simulink library "lib_lowphy"  (R2023b)
settings: Solver=VariableStepAuto  StartTime=0.0  StopTime=10.0  RelTol=1e-3
undefined symbols (not defined in the file or in its folder): AdvDSPBChannelOutDisplay, AdvDSPBDMemDisplay, AdvDSPBInDisplay, AdvDSPBOutDisplay, dpoly, dspba, dspba_ChannelInVis, dspba_ChannelOutVis, dspba_internal_get_channel_ports, evalAionMaskParam, fft_tb_in, ifft_tb_in, latency, latencyCorrection, max_FFTStages, max_NSubcarriers, primtype, UseDontCare, value
libraries: DSPBAPrim x637, DSPBAControl x55, $bdroot x16, DSPBAModelBus x12, DSPBAUtilities x6, DSPBABase x5, DSPBAWaveformSynth x4, DspbAdvFftLibrary x3, DSPBAVectorUtil x2, DspbAdvVfftPrefix x1
(part 1 of 9)
settings Model: Creator=manjukri  LastModifiedBy=5g
settings DebuggingCC: UnconnectedInputMsg=warning  UnconnectedOutputMsg=warning  UnconnectedLineMsg=warning
settings ModelReferenceCC: EnableRefExpFcnMdlSchedulingChecks=on
settings RTWCC: DLArmComputeVersion=19.05

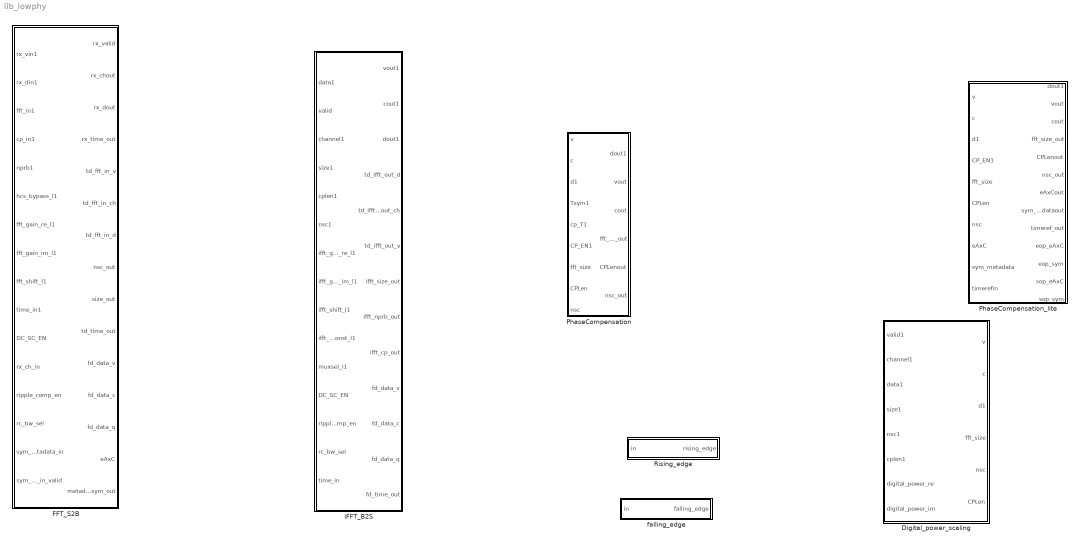
== system lib_lowphy ==
  Digital_power_scaling : Subsystem
  FFT_S2B : Subsystem  mask{FFTmaxsize=12, FFTminsize=9, FFTstages=12, Rx_scaling=2^-12, AxCdelay=288, NCO_addr_offset=0, rc_out_frac=11}
      mask prompts: FFTmaxsize "FFT max size"; FFTminsize "FFT Min Size"; FFTstages "FFT stages"; Rx_scaling "Fractional Precision output of FFT"; AxCdelay "delay between AxC block output"; NCO_addr_offset "NCO address offset (length =4)"; rc_out_frac "enter_ripple_comp_out_frac_bits"
      mask init:
      | fsmpaths
      | 
      | 
      | 
      | 
      | %% FFT configuration
      | dspb_fft_multichannel.IFFT = false;
      | dspb_fft_multichannel.minsize = FFTminsize;
      | dspb_fft_multichannel.maxsize = FFTmaxsize;
      | dspb_fft_multichannel.N = FFTstages;
      | dspb_fft_multichannel.subchannels = 1; % must be a power of 2
      | dspb_fft_multichannel.FFTsize = 2^dspb_fft_multichannel.N;
      | dspb_fft_multichannel.blockSize = dspb_fft_multichannel.subchannels * dspb_fft_multichannel.FFTsize;
      | 
      | %% Data widths
      | dspb_fft_multichannel.InputType   = fixdt(1,16,13);
      | dspb_fft_multichannel.TwiddleType = fixdt(1,16,15);
      | 
      | dspb_fft_multichannel.Phase_Inversion_l1   = 15;
      | dspb_fft_multichannel.fft_gain_offset_l1   = 1;
      | dspb_fft_multichannel.fft_gain_value       = 1;
      | dspb_fft_multichannel.HCS_Bypass_offset_l1 = 2;
      | dspb_fft_multichannel.HCS_Bypass_value     = 1;
      | 
      | dspb_fft_multichannel.Phase_Inversion_l2   = 20;
      | dspb_fft_multichannel.fft_gain_offset_l2   = 3;
      | dspb_fft_multichannel.HCS_Bypass_offset_l2 = 4;
      | dspb_fft_multichannel.sclowerselect_l2 =5;
      | dspb_fft_multichannel.ClockRate	=  491.52;
      | 
      | 
      | %% Pruning options
      | %dspb_fft_multichannel.TypeStrings0 = some user-defined strategy
      | 
      | dspb_fft_multichannel.TypeStrings1 = ...
      |     dspba.fft.full_wordgrowth(true, false, dspb_fft_multichannel.N,...
      |         dspb_fft_multichannel.InputType, dspb_fft_multichannel.TwiddleType);
      | 
      | dspb_fft_multichannel.TypeStrings2 = ...
      |     dspba.fft.mild_pruning(true, false, dspb_fft_multichannel.N,...
      |         dspb_fft_multichannel.InputType, dspb_fft_multichannel.TwiddleType); 
      | 
      | dspb_fft_multichannel.TypeStrings3 = ...
      |     dspba.fft.prune_to_width(19, true, false, dspb_fft_multichannel.N,...
      |         dspb_fft_multichannel.InputType, dspb_fft_multichannel.TwiddleType);
      | 
      | dspb_fft_multichannel.TypeStrings = dspb_fft_multichannel.TypeStrings1;
      | 
      | 
      | 
      | FeedbackDelay1=12;
  PhaseCompensation : Subsystem  mask{Tc=1/122.88e6, CP_1=352, CP_2=288, PhaseGen_TXRX=0, Op_frac_scaling=2^-14}
      mask prompts: Tc "Sample time"; CP_1 "CP Sample Length Sym 0"; CP_2 "CP Sample Length Sym 1-13"; PhaseGen_TXRX "Phase Sign (1= -ve phase for Tx , 0 = +ve phase for Rx)"; Op_frac_scaling "Output Fractional scaling"
      mask init:
      | %% MM Register Setting
      | MMoffset.F1_regLSB = 0;
      | MMoffset.F1_regMSB = 1;
      | MMoffset.Enable_reg1 = 2;
      | MMoffset.PhaseGen_reg = 3;
      | 
      | 
      | 
      | 
      | cordic_gain = 1.646760257865452963193594414453;
      | 
      | 
      | 
      | CPSample_Vector_LUT = [ CP_1*Tc CP_2*Tc*ones(1,13)]*1e9; % t is given in ns as F is given in Ghz
      | 
      | 
      | 
      | 
      | 
      | 
      | dspb_ifft_multichannel.ClockRate=491.52;
  PhaseCompensation_lite : Subsystem  mask{Tc=1/122.88e6, CP_1=352, CP_2=288, PhaseGen_TXRX=0, Op_frac_scaling=2^-14, reg_mem_offset_rf_freq=0, reg_mem_offset_Phase_comp_enable=1, reg_mem_offset_tx_rx_sel=2}
      mask prompts: Tc "Sample time"; CP_1 "CP Sample Length Sym 0"; CP_2 "CP Sample Length Sym 1-13"; PhaseGen_TXRX "Phase Sign (1= -ve phase for Tx , 0 = +ve phase for Rx)"; Op_frac_scaling "Output Fractional scaling"; reg_mem_offset_rf_freq "Address offset of register holding RF Frequency"; reg_mem_offset_Phase_comp_enable "Address offset of register holding Phase Compensation enable"; reg_mem_offset_tx_rx_sel "Address offset of register holding  Tx Rx Selection"
      mask init:
      | %% MM Register Setting
      | MMoffset.F1_regLSB = 0;
      | MMoffset.F1_regMSB = 1;
      | MMoffset.Enable_reg1 = 2;
      | MMoffset.PhaseGen_reg = 3;
      | 
      | 
      | 
      | 
      | cordic_gain = 1.646760257865452963193594414453;
      | 
      | 
      | 
      | CPSample_Vector_LUT = [ CP_1*Tc CP_2*Tc*ones(1,13)]*1e9; % t is given in ns as F is given in Ghz
      | 
      | 
      | 
      | 
      | 
      | 
      | dspb_ifft_multichannel.ClockRate=491.52;
      | 
      | %Tsym_reinterpret_LUT=[ 2.87272135416667e-06 3.85498046875000e-05 7.42268880208333e-05 0.000109903971354167 0.000145581054687500 0.000181258138020833 0.000216935221354167 0.000252612304687500 0.000288289388020833 0.000323966471354167 0.000359643554687500 0.000395320638020833 0.000430997721354167 0.000466674804687500 ]*1e9;
  Rising_edge : Subsystem
      mask init:
      | fsmpaths
  falling_edge : Subsystem
      mask init:
      | fsmpaths
  iFFT_B2S : Subsystem  mask{iFFTmaxsize=12, iFFTminsize=9, iFFTstages=12, Tx_scaling=2^-14, Bw_Delay_en=1, rc_out_frac=12}
      mask prompts: iFFTmaxsize "iFFT Maxsize"; iFFTminsize "iFFT Minsize"; iFFTstages "iFFT Stages"; Tx_scaling "Fractional precision output of iFFT_B2B"; Bw_Delay_en "Delay Alignment for Bandwidth (60 & 100MHz)"; rc_out_frac "ripple compensation out fractional value"
      mask init:
      | %% IFFT configuration
      | dspb_ifft_multichannel.IFFT = true;
      | dspb_ifft_multichannel.minsize = iFFTminsize;
      | dspb_ifft_multichannel.maxsize = iFFTmaxsize;
      | dspb_ifft_multichannel.N = iFFTstages;
      | dspb_ifft_multichannel.subchannels = 1; % must be a power of 2
      | dspb_ifft_multichannel.FFTsize = 2^dspb_ifft_multichannel.N;
      | dspb_ifft_multichannel.blockSize = dspb_ifft_multichannel.subchannels * dspb_ifft_multichannel.FFTsize;
      | 
      | %% Data widths
      | dspb_ifft_multichannel.InputType   = fixdt(1,16,rc_out_frac);
      | dspb_ifft_multichannel.TwiddleType = fixdt(1,16,15);
      | 
      | 
      | 
      | 
      | %% Pruning options
      | %dspb_ifft_multichannel.TypeStrings0 = some user-defined strategy
      | 
      | dspb_ifft_multichannel.TypeStrings1 = ...
      |     dspba.fft.full_wordgrowth(true, false, dspb_ifft_multichannel.N,...
      |         dspb_ifft_multichannel.InputType, dspb_ifft_multichannel.TwiddleType);
      | 
      | dspb_ifft_multichannel.TypeStrings2 = ...
      |     dspba.fft.mild_pruning(true, false, dspb_ifft_multichannel.N,...
      |         dspb_ifft_multichannel.InputType, dspb_ifft_multichannel.TwiddleType);
      | 
      | dspb_ifft_multichannel.TypeStrings3 = ...
      |     dspba.fft.prune_to_width(19, true, false, dspb_ifft_multichannel.N,...
      |         dspb_ifft_multichannel.InputType, dspb_ifft_multichannel.TwiddleType);
      | 
      | dspb_ifft_multichannel.TypeStrings = dspb_ifft_multichannel.TypeStrings1;
      | 
      | %%
      |  CP_ProcessingDelay =30;
      | SampleReg_pipelineDelay = 14;
      | max_FFTStages=iFFTstages;
      | max_NSubcarriers=3276;

== system lib_lowphy/Digital_power_scaling ==
  valid1 : Inport
  channel1 : Inport  Port=2
  data1 : Inport  Port=3
  size1 : Inport  Port=4
  nsc1 : Inport  Port=5
  cplen1 : Inport  Port=6
  digital_power_re : Inport  Port=7
  digital_power_im : Inport  Port=8
  Mult : DSPBAPrim/Mult  primtype=mult  nInputs=2  nOutputs=1  omode=Inherit via internal rule  otype=sfix(16)  scale=2^-15  rndmethod=Unbiased  factor=1  satmethod=Symmetric  shift_vec=[0 1 2 -1]  value=0  inPortNames=[' '; ' ';]  outPortNames=[' ']  dspbaimage=dspba_prim.svg  text=fprintf('X');  style=Optimised  visibilities=8+2^18+2^19  floatPrecision=float32_m23  floatRounding=correct  advOptions=[]  version=20211007
  Real-Imag to Complex : RealImagToComplex
  Scale1 : DSPBAPrim/Convert  primtype=convert  nInputs=1  nOutputs=1  omode=Specify via dialog  otype=sfix(16)  scale=2^-15  rndmethod=Biased  factor=1  satmethod=Symmetric  shift_vec=[0 1 2 -1]  value=round([0:255]/17)  inPortNames=[' '; ' ';]  outPortNames=[' '; 'c']  dspbaimage=dspba_prim_wide.svg  text=fprintf('convert');  style=Optimised  visibilities=8+64+256+2^17  clipdetect=off  floatPrecision=float32_m23  advOptions=[]  version=20211007
  SynthesisInfo : DSPBAPrim/SynthesisInfo  primtype=synthinfo  nInputs=0  nOutputs=0  omode=Inherit via internal rule  otype=sfix(16)  scale=2^-15  rndmethod=Truncate  factor=1  satmethod=Symmetric  shift_vec=[0 1 2 -1]  value=99  inPortNames=[' '; ' ';]  outPortNames=[' ']  dspbaimage=dspba_prim_ctrl.jpg  text=fprintf('Style=%s', style);  style=Scheduled  visibilities=2^17+2^18+2^19+2^20+2^21+2^22+2^23+2^24  constraintPair=None  constraintRelation=>  constraintLimit=2  modelRefSign=+  modelRef=''  showSchedule=off  simulationMode=Use Global Value  resetMinimization=Conditional - On for ChannelIn/Out only  version=20220106
  channel_DPS1_in : DSPBAPrim/ChannelIn  primtype=channelin  nInputs=dspba_internal_get_channel_ports(gcb)  nOutputs=dspba_internal_get_channel_ports(gcb)  omode=Inherit via internal rule  otype=sfix(16)  scale=2^-15  rndmethod=Unbiased  factor=1  satmethod=Symmetric  shift_vec=[0 1 2 -1]  value=6  inPortNames=['v'; 'c'; '0'; '1'; '2'; '3'; '4'; '5'; '6'; '7'; '8'; '9'; 'A'; 'B'; 'D'; 'E'; 'F'; 'G'; 'H'; 'I'; 'J'; 'K'; 'L'; 'M'; 'N'; 'O'; 'P'; 'Q'; 'R'; 'S'; 'T'; 'U'; 'W'; 'X'; 'Y'; 'Z']  outPortNames=['v'; 'c'; '0'; '1'; '2'; '3'; '4'; '5'; '6'; '7'; '8'; '9'; 'A'; 'B'; 'D'; 'E'; 'F'; 'G'; 'H'; 'I'; 'J'; 'K'; 'L'; 'M'; 'N'; 'O'; 'P'; 'Q'; 'R'; 'S'; 'T'; 'U'; 'W'; 'X'; 'Y'; 'Z']  dspbaimage=dspba_prim_channel_tall.svg  text=fprintf('In');  style=Optimised  dataSignals=6  foldingEnabled=off  channels=1  sampleRate=200  packetBeginPresent=off  packetBeginEnabled=off  visibilities=dspba_ChannelInVis(gcb)  latencyCorrection=0  scheduleOrigin=on  version=20211214
  channel_DPS1_out : DSPBAPrim/ChannelOut  primtype=channelout  nInputs=dspba_internal_get_channel_ports(gcb)  nOutputs=dspba_internal_get_channel_ports(gcb)  omode=Inherit via internal rule  otype=sfix(16)  scale=2^-15  rndmethod=Unbiased  factor=1  satmethod=Symmetric  shift_vec=[0 1 2 -1]  value=4  inPortNames=['v'; 'c'; '0'; '1'; '2'; '3'; '4'; '5'; '6'; '7'; '8'; '9'; 'A'; 'B'; 'D'; 'E'; 'F'; 'G'; 'H'; 'I'; 'J'; 'K'; 'L'; 'M'; 'N'; 'O'; 'P'; 'Q'; 'R'; 'S'; 'T'; 'U'; 'W'; 'X'; 'Y'; 'Z']  outPortNames=['v'; 'c'; '0'; '1'; '2'; '3'; '4'; '5'; '6'; '7'; '8'; '9'; 'A'; 'B'; 'D'; 'E'; 'F'; 'G'; 'H'; 'I'; 'J'; 'K'; 'L'; 'M'; 'N'; 'O'; 'P'; 'Q'; 'R'; 'S'; 'T'; 'U'; 'W'; 'X'; 'Y'; 'Z']  dspbaimage=dspba_prim_channel_tall.svg  text=fprintf('Out%s', AdvDSPBChannelOutDisplay(latency));  style=Optimised  dataSignals=4  foldingEnabled=off  channels=1  sampleRate=200  packetBeginPresent=off  packetBeginEnabled=off  visibilities=dspba_ChannelOutVis(gcb)  latency=8  latencyCorrection=0  version=20211214
  v : Outport
  c : Outport  Port=2
  d1 : Outport  Port=3
  fft_size : Outport  Port=4
  nsc : Outport  Port=5
  CPLen : Outport  Port=6
  wires:
  valid1/1 -> channel_DPS1_in/1
  channel1/1 -> channel_DPS1_in/2
  data1/1 -> channel_DPS1_in/3
  channel_DPS1_out/3 -> d1/1
  channel_DPS1_out/4 -> fft_size/1
  channel_DPS1_out/2 -> c/1
  channel_DPS1_out/1 -> v/1
  size1/1 -> channel_DPS1_in/4
  nsc1/1 -> channel_DPS1_in/5
  channel_DPS1_out/5 -> nsc/1
  cplen1/1 -> channel_DPS1_in/6
  digital_power_re/1 -> channel_DPS1_in/7
  digital_power_im/1 -> channel_DPS1_in/8
  channel_DPS1_in/7 -> Real-Imag to Complex/1
  channel_DPS1_in/8 -> Real-Imag to Complex/2
  channel_DPS1_in/3 -> Mult/1
  Real-Imag to Complex/1 -> Mult/2
  channel_DPS1_in/4 -> channel_DPS1_out/4
  channel_DPS1_in/5 -> channel_DPS1_out/5
  channel_DPS1_in/6 -> channel_DPS1_out/6
  channel_DPS1_in/1 -> channel_DPS1_out/1
  channel_DPS1_in/2 -> channel_DPS1_out/2
  Scale1/1 -> channel_DPS1_out/3
  Mult/1 -> Scale1/1
  channel_DPS1_out/6 -> CPLen/1

== system lib_lowphy/FFT_S2B ==
  rx_vin1 : Inport
  rx_din1 : Inport  Port=2
  fft_in1 : Inport  Port=3
  cp_in1 : Inport  Port=4
  nprb1 : Inport  Port=5
  hcs_bypass_l1 : Inport  Port=6
  fft_gain_re_l1 : Inport  Port=7
  fft_gain_im_l1 : Inport  Port=8
  fft_shift_l1 : Inport  Port=9
  time_in1 : Inport  Port=10
  DC_SC_EN : Inport  Port=11
  rx_ch_in : Inport  Port=12
  ripple_comp_en : Inport  Port=13
  rc_bw_sel : Inport  Port=14
  sym_metadata_in : Inport  Port=15
  sym_metadata_in_valid : Inport  Port=16
  CPRemoval : Subsystem
  Const : DSPBAPrim/Const  primtype=const  nInputs=0  nOutputs=1  omode=Specify via dialog  otype=fixdt(0,3,0)  scale=0  rndmethod=Unbiased  factor=1  satmethod=Symmetric  shift_vec=[0 1 2 -1]  value=2  inPortNames=['+'; '+';]  outPortNames=[' ']  dspbaimage=dspba_prim.svg  text=fprintf('%s', num2str(value));  style=Optimised  visibilities=8 + 1024  floatPrecision=float32_m23  warnSaturation=on  version=20211007  SampleTime=inf
  SignalProcessing : Subsystem
  rx_valid : Outport
  rx_chout : Outport  Port=2
  rx_dout : Outport  Port=3
  rx_time_out : Outport  Port=4
  td_fft_in_v : Outport  Port=5
  td_fft_in_ch : Outport  Port=6
  td_fft_in_d : Outport  Port=7
  nsc_out : Outport  Port=8
  size_out : Outport  Port=9
  td_time_out : Outport  Port=10
  fd_data_v : Outport  Port=11
  fd_data_c : Outport  Port=12
  fd_data_q : Outport  Port=13
  eAxC : Outport  Port=14
  metadata_sym_out : Outport  Port=15
  wires:
  SignalProcessing/10(td_time_out) -> td_time_out/1
  SignalProcessing/9(size_out) -> size_out/1
  CPRemoval/3(dout) -> SignalProcessing/3(din)
  CPRemoval/1("vout ") -> SignalProcessing/4(sync), SignalProcessing/1(fft_v_in)
  nprb1/1 -> CPRemoval/8(nprb_in)
  rc_bw_sel/1 -> SignalProcessing/14(rc_bw_sel)
  SignalProcessing/2(rxnat_chout) -> rx_chout/1
  CPRemoval/2(cout) -> SignalProcessing/2(cin)
  CPRemoval/5(nprb_out) -> SignalProcessing/5(nsc)
  CPRemoval/4(time_out) -> SignalProcessing/7(SFNin)
  Const/1 -> CPRemoval/6(NumAxc)
  fft_in1/1 -> CPRemoval/5(fftlen)
  CPRemoval/6(fft_size_out) -> SignalProcessing/6(size)
  rx_ch_in/1 -> CPRemoval/3(cin)
  SignalProcessing/6(td_fft_in_ch) -> td_fft_in_ch/1
  rx_vin1/1 -> CPRemoval/2(vin)
  rx_din1/1 -> CPRemoval/1(datain)
  SignalProcessing/1(rxnat_vout) -> rx_valid/1
  SignalProcessing/3(rxnat_dout) -> rx_dout/1
  fft_gain_im_l1/1 -> SignalProcessing/9(fft_gain_im)
  hcs_bypass_l1/1 -> SignalProcessing/10(hcs_bypass)
  SignalProcessing/7(td_fft_in_d) -> td_fft_in_d/1
  fft_shift_l1/1 -> SignalProcessing/11(fft_shift)
  time_in1/1 -> CPRemoval/7(time_in)
  fft_gain_re_l1/1 -> SignalProcessing/8(fft_gain_re)
  DC_SC_EN/1 -> SignalProcessing/12(DC_SC_EN)
  ripple_comp_en/1 -> SignalProcessing/13(ripple_comp_en)
  cp_in1/1 -> CPRemoval/4(CPlen)
  SignalProcessing/4(rx_time_out) -> rx_time_out/1
  SignalProcessing/5(td_fft_in_v) -> td_fft_in_v/1
  SignalProcessing/8(nsc_out) -> nsc_out/1
  SignalProcessing/11(fd_v) -> fd_data_v/1
  SignalProcessing/12(fd_c) -> fd_data_c/1
  SignalProcessing/13(fd_q) -> fd_data_q/1
  sym_metadata_in/1 -> CPRemoval/9(sym_metadata_in)
  sym_metadata_in_valid/1 -> CPRemoval/10(sym_metadata_in_valid)
  CPRemoval/7(eAxC_no) -> SignalProcessing/15(eAxc)
  CPRemoval/8(sym_metadata) -> SignalProcessing/16(sym_metadata)
  SignalProcessing/14(eAxC) -> eAxC/1
  SignalProcessing/15(metadata_sym_out) -> metadata_sym_out/1

== system lib_lowphy/PhaseCompensation ==
  v : Inport
  c : Inport  Port=2
  d1 : Inport  Port=3
  Tsym1 : Inport  Port=4
  cp_T1 : Inport  Port=5
  CP_EN1 : Inport  Port=6
  fft_size : Inport  Port=7
  CPLen : Inport  Port=8
  nsc : Inport  Port=9
  ComplexMixer : Subsystem
  PhasorGenerate : Subsystem
  Real-Imag to Complex : RealImagToComplex
  To Workspace : ToWorkspace  VariableName=PhaseGenDout  SaveFormat=Timeseries  SampleTime=-1
  To Workspace1 : ToWorkspace  VariableName=PhaseGenValidout  SaveFormat=Timeseries  SampleTime=-1
  To Workspace2 : ToWorkspace  VariableName=PhaseGenCosSin  SaveFormat=Timeseries  SampleTime=-1
  To Workspace3 : ToWorkspace  VariableName=PhFinalDout  SaveFormat=Timeseries  SampleTime=-1
  To Workspace4 : ToWorkspace  VariableName=PhFinalValid  SaveFormat=Timeseries  SampleTime=-1
  dout1 : Outport
  vout : Outport  Port=2
  cout : Outport  Port=3
  fft_size_out : Outport  Port=4
  CPLenout : Outport  Port=5
  nsc_out : Outport  Port=6
  wires:
  PhasorGenerate/3(cout) -> ComplexMixer/3(cin)
  PhasorGenerate/4(sin) -> Real-Imag to Complex/2, ComplexMixer/4(sin)
  ComplexMixer/1(dout1) -> To Workspace3/1, dout1/1
  PhasorGenerate/5(cos) -> ComplexMixer/5(cos), Real-Imag to Complex/1
  ComplexMixer/3(cout) -> cout/1
  PhasorGenerate/1(dout1) -> To Workspace/1, ComplexMixer/1(din1)
  d1/1 -> PhasorGenerate/3(d1)
  PhasorGenerate/7(CPLenout) -> CPLenout/1
  fft_size/1 -> PhasorGenerate/7(fft_size)
  PhasorGenerate/8(nsc_out) -> nsc_out/1
  PhasorGenerate/2(vout) -> To Workspace1/1, ComplexMixer/2(vin)
  ComplexMixer/2(vout) -> To Workspace4/1, vout/1
  nsc/1 -> PhasorGenerate/9(nsc)
  c/1 -> PhasorGenerate/2(c)
  CP_EN1/1 -> PhasorGenerate/6(CP_EN1)
  PhasorGenerate/6(fft_size_out) -> fft_size_out/1
  v/1 -> PhasorGenerate/1(v)
  cp_T1/1 -> PhasorGenerate/5(cp_T1)
  CPLen/1 -> PhasorGenerate/8(CPLen)
  Tsym1/1 -> PhasorGenerate/4(Tsym1)
  Real-Imag to Complex/1 -> To Workspace2/1

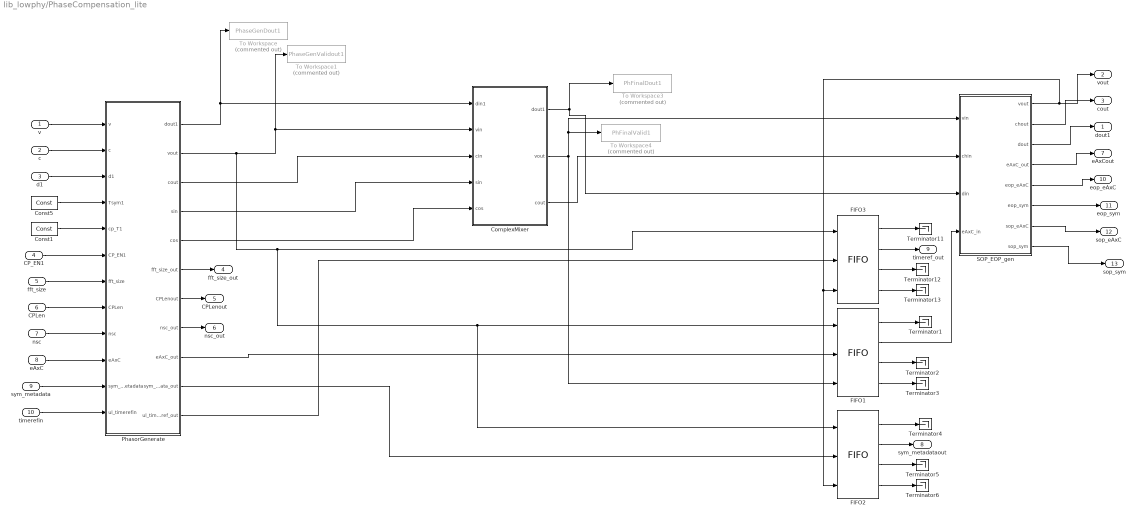
== system lib_lowphy/PhaseCompensation_lite ==
  v : Inport
  c : Inport  Port=2
  d1 : Inport  Port=3
  CP_EN1 : Inport  Port=4
  fft_size : Inport  Port=5
  CPLen : Inport  Port=6
  nsc : Inport  Port=7
  eAxC : Inport  Port=8
  sym_metadata : Inport  Port=9
  timerefin : Inport  Port=10
  ComplexMixer : Subsystem
  Const1 : DSPBAPrim/Const  primtype=const  nInputs=0  nOutputs=1  omode=Specify via dialog  otype=sfix(16)  scale=2^-15  rndmethod=Unbiased  factor=1  satmethod=Symmetric  shift_vec=[0 1 2 -1]  value=0  inPortNames=['+'; '+';]  outPortNames=[' ']  dspbaimage=dspba_prim.svg  text=fprintf('%s', num2str(value));  style=Optimised  visibilities=8 + 1024  floatPrecision=float32_m23  warnSaturation=on  version=20211007  SampleTime=inf
  Const5 : DSPBAPrim/Const  primtype=const  nInputs=0  nOutputs=1  omode=Specify via dialog  otype=sfix(16)  scale=2^-15  rndmethod=Unbiased  factor=1  satmethod=Symmetric  shift_vec=[0 1 2 -1]  value=0  inPortNames=['+'; '+';]  outPortNames=[' ']  dspbaimage=dspba_prim.svg  text=fprintf('%s', num2str(value));  style=Optimised  visibilities=8 + 1024  floatPrecision=float32_m23  warnSaturation=on  version=20211007  SampleTime=inf
  FIFO1 : DSPBAPrim/FIFO  primtype=fifo  nInputs=3  nOutputs=4  omode=Inherit via internal rule  otype=sfix(16)  scale=2^-15  rndmethod=Unbiased  factor=1  satmethod=Symmetric  shift_vec=[0 1 2 -1]  value=[128 4 64]  inPortNames=['w'; 'd'; 'r'; 'f']  outPortNames=['v'; 'q'; 't'; 'f']  dspbaimage=dspba_prim_tall.svg  text=fprintf('fifo');  style=Optimised  visibilities=263168  version=20211007  user_sclr=off
  FIFO2 : DSPBAPrim/FIFO  primtype=fifo  nInputs=3  nOutputs=4  omode=Inherit via internal rule  otype=sfix(16)  scale=2^-15  rndmethod=Unbiased  factor=1  satmethod=Symmetric  shift_vec=[0 1 2 -1]  value=[64 4 16]  inPortNames=['w'; 'd'; 'r'; 'f']  outPortNames=['v'; 'q'; 't'; 'f']  dspbaimage=dspba_prim_tall.svg  text=fprintf('fifo');  style=Optimised  visibilities=263168  version=20211007  user_sclr=off
  FIFO3 : DSPBAPrim/FIFO  primtype=fifo  nInputs=3  nOutputs=4  omode=Inherit via internal rule  otype=sfix(16)  scale=2^-15  rndmethod=Unbiased  factor=1  satmethod=Symmetric  shift_vec=[0 1 2 -1]  value=[64 4 16]  inPortNames=['w'; 'd'; 'r'; 'f']  outPortNames=['v'; 'q'; 't'; 'f']  dspbaimage=dspba_prim_tall.svg  text=fprintf('fifo');  style=Optimised  visibilities=263168  version=20211007  user_sclr=off
  PhasorGenerate : Subsystem
  SOP_EOP_gen : Subsystem
  Terminator{1..6,11..13} (9 alike) : Terminator
  To Workspace : ToWorkspace  Commented=on  VariableName=PhaseGenDout1  SaveFormat=Timeseries  SampleTime=-1
  To Workspace1 : ToWorkspace  Commented=on  VariableName=PhaseGenValidout1  SaveFormat=Timeseries  SampleTime=-1
  To Workspace3 : ToWorkspace  Commented=on  VariableName=PhFinalDout1  SaveFormat=Timeseries  SampleTime=-1
  To Workspace4 : ToWorkspace  Commented=on  VariableName=PhFinalValid1  SaveFormat=Timeseries  SampleTime=-1
  dout1 : Outport
  vout : Outport  Port=2
  cout : Outport  Port=3
  fft_size_out : Outport  Port=4
  CPLenout : Outport  Port=5
  nsc_out : Outport  Port=6
  eAxCout : Outport  Port=7
  sym_metadataout : Outport  Port=8
  timeref_out : Outport  Port=9
  eop_eAxC : Outport  Port=10
  eop_sym : Outport  Port=11
  sop_eAxC : Outport  Port=12
  sop_sym : Outport  Port=13
  wires:
  FIFO1/3 -> Terminator2/1
  PhasorGenerate/6(fft_size_out) -> fft_size_out/1
  SOP_EOP_gen/2(chout) -> cout/1
  FIFO2/4 -> Terminator6/1
  SOP_EOP_gen/3(dout) -> dout1/1
  SOP_EOP_gen/8(sop_sym) -> sop_sym/1
  FIFO2/1 -> Terminator4/1
  PhasorGenerate/8(nsc_out) -> nsc_out/1
  FIFO2/3 -> Terminator5/1
  FIFO3/3 -> Terminator12/1
  Const1/1 -> PhasorGenerate/5(cp_T1)
  ComplexMixer/2(vout) -> FIFO1/3, SOP_EOP_gen/1(vin), To Workspace4/1
  PhasorGenerate/11(ul_timeref_out) -> FIFO3/2
  ComplexMixer/1(dout1) -> SOP_EOP_gen/3(din), To Workspace3/1
  SOP_EOP_gen/4(eAxC_out) -> eAxCout/1
  PhasorGenerate/5(cos) -> ComplexMixer/5(cos)
  PhasorGenerate/3(cout) -> ComplexMixer/3(cin)
  CP_EN1/1 -> PhasorGenerate/6(CP_EN1)
  PhasorGenerate/7(CPLenout) -> CPLenout/1
  PhasorGenerate/4(sin) -> ComplexMixer/4(sin)
  eAxC/1 -> PhasorGenerate/10(eAxC)
  nsc/1 -> PhasorGenerate/9(nsc)
  FIFO1/1 -> Terminator1/1
  PhasorGenerate/1(dout1) -> To Workspace/1, ComplexMixer/1(din1)
  timerefin/1 -> PhasorGenerate/12(ul_timerefin)
  FIFO1/2 -> SOP_EOP_gen/4(eAxC_in)
  c/1 -> PhasorGenerate/2(c)
  ComplexMixer/3(cout) -> SOP_EOP_gen/2(chin)
  sym_metadata/1 -> PhasorGenerate/11(sym_metadata)
  FIFO3/4 -> Terminator13/1
  SOP_EOP_gen/7(sop_eAxC) -> sop_eAxC/1
  SOP_EOP_gen/1(vout) -> vout/1, FIFO2/3, FIFO3/3
  PhasorGenerate/9(eAxC_out) -> FIFO1/2
  Const5/1 -> PhasorGenerate/4(Tsym1)
  FIFO3/1 -> Terminator11/1
  fft_size/1 -> PhasorGenerate/7(fft_size)
  FIFO1/4 -> Terminator3/1
  CPLen/1 -> PhasorGenerate/8(CPLen)
  d1/1 -> PhasorGenerate/3(d1)
  PhasorGenerate/10(sym_metadata_out) -> FIFO2/2
  FIFO3/2 -> timeref_out/1
  PhasorGenerate/2(vout) -> FIFO2/1, FIFO1/1, FIFO3/1, To Workspace1/1, ComplexMixer/2(vin)
  SOP_EOP_gen/5(eop_eAxC) -> eop_eAxC/1
  SOP_EOP_gen/6(eop_sym) -> eop_sym/1
  FIFO2/2 -> sym_metadataout/1
  v/1 -> PhasorGenerate/1(v)

== system lib_lowphy/Rising_edge ==
  in : Inport
  Const : DSPBAPrim/Const  primtype=const  nInputs=0  nOutputs=1  omode=Specify via dialog  otype=ufix(1)  scale=0  rndmethod=Unbiased  factor=1  satmethod=Symmetric  shift_vec=[0 1 2 -1]  value=1  inPortNames=['+'; '+';]  outPortNames=[' ']  dspbaimage=dspba_prim.svg  text=fprintf('%s', num2str(value));  style=Optimised  visibilities=8 + 1024 + 2^18 + 2^20  floatPrecision=float32_m23  warnSaturation=on  version=20211007  SampleTime=inf
  Convert : DSPBAPrim/Convert  primtype=convert  nInputs=1  nOutputs=1  omode=Specify via dialog  otype=ufix(1)  scale=0  rndmethod=Unbiased  factor=1  satmethod=None  shift_vec=[0 1 2 -1]  value=round([0:255]/17)  inPortNames=[' '; ' ';]  outPortNames=[' '; 'c']  dspbaimage=dspba_prim_wide.svg  text=fprintf('convert');  style=Optimised  visibilities=8+64+256+2^17  clipdetect=off  floatPrecision=float32_m23  advOptions=[]  version=20211007
  Finite State Machine : DSPBAUtilities/Finite State Machine  desc_file=fsm_control_rising_edge.fsm  latency=0  simulationMode=Bit And Cycle Accurate  finiteStateMachine=on
  GPIn : DSPBAPrim/GPIn  Commented=through  primtype=gpin  nInputs=evalAionMaskParam(gcb,'value',1)  nOutputs=evalAionMaskParam(gcb,'value',1)  omode=Inherit via internal rule  otype=sfix(16)  scale=2^-15  rndmethod=Unbiased  factor=1  satmethod=Symmetric  shift_vec=[0 1 2 -1]  value=1  inPortNames=[' ' ' ' ' ' ' ' ' ' ' ' ' ' ' ' ' ' ' ' ' ' ' ' ' ' ' ' ' ' ' ' ' ' ' ' ' ' ' ' ' ' ' ' ' ' ' ' ' ' ' ' ' ' ' ' ' ' ' ' ' ' ' ' ' ' ' ' ' ']'  outPortNames=[' ' ' ' ' ' ' ' ' ' ' ' ' ' ' ' ' ' ' ' ' ' ' ' ' ' ' ' ' ' ' ' ' ' ' ' ' ' ' ' ' ' ' ' ' ' ' ' ' ' ' ' ' ' ' ' ' ' ' ' ' ' ' ' ' ' ' ' ' ']'  dspbaimage=dspba_prim_channel_tall.svg  text=fprintf('GPIn%s', AdvDSPBInDisplay(latencyCorrection));  style=Optimised  visibilities=1024  latencyCorrection=0  scheduleOrigin=on  version=20211214
  GPOut : DSPBAPrim/GPOut  Commented=through  primtype=gpout  nInputs=evalAionMaskParam(gcb,'value',1)  nOutputs=evalAionMaskParam(gcb,'value',1)  omode=Inherit via internal rule  otype=sfix(16)  scale=2^-15  rndmethod=Unbiased  factor=1  satmethod=Symmetric  shift_vec=[0 1 2 -1]  value=1  inPortNames=[' ' ' ' ' ' ' ' ' ' ' ' ' ' ' ' ' ' ' ' ' ' ' ' ' ' ' ' ' ' ' ' ' ' ' ' ' ' ' ' ' ' ' ' ' ' ' ' ' ' ' ' ' ' ' ' ' ' ' ' ' ' ' ' ' ' ' ' ' ']'  outPortNames=[' ' ' ' ' ' ' ' ' ' ' ' ' ' ' ' ' ' ' ' ' ' ' ' ' ' ' ' ' ' ' ' ' ' ' ' ' ' ' ' ' ' ' ' ' ' ' ' ' ' ' ' ' ' ' ' ' ' ' ' ' ' ' ' ' ' ' ' ' ']'  dspbaimage=dspba_prim_channel_tall.svg  text=fprintf('GPOut%s', AdvDSPBOutDisplay(latency, latencyCorrection));  style=Optimised  visibilities=1024  latency=0  latencyCorrection=0  version=20211214
  SynthesisInfo : DSPBAPrim/SynthesisInfo  Commented=on  primtype=synthinfo  nInputs=0  nOutputs=0  omode=Inherit via internal rule  otype=sfix(16)  scale=2^-15  rndmethod=Truncate  factor=1  satmethod=Symmetric  shift_vec=[0 1 2 -1]  value=99  inPortNames=[' '; ' ';]  outPortNames=[' ']  dspbaimage=dspba_prim_ctrl.jpg  text=fprintf('Style=%s', style);  style=Scheduled  visibilities=2^17+2^18+2^19+2^20+2^21+2^22+2^23+2^24  constraintPair=GPIn to GPOut  constraintRelation==  constraintLimit=0  modelRefSign=+  modelRef=''  showSchedule=off  simulationMode=Use Global Value  resetMinimization=Conditional - On for ChannelIn/Out only  version=20220106
  rising_edge : Outport
  wires:
  GPIn/1 -> Convert/1
  Finite State Machine/1 -> GPOut/1
  Const/1 -> Finite State Machine/1
  GPOut/1 -> rising_edge/1
  in/1 -> GPIn/1
  Convert/1 -> Finite State Machine/2

== system lib_lowphy/falling_edge ==
  in : Inport
  Const : DSPBAPrim/Const  primtype=const  nInputs=0  nOutputs=1  omode=Specify via dialog  otype=ufix(1)  scale=0  rndmethod=Unbiased  factor=1  satmethod=Symmetric  shift_vec=[0 1 2 -1]  value=1  inPortNames=['+'; '+';]  outPortNames=[' ']  dspbaimage=dspba_prim.svg  text=fprintf('%s', num2str(value));  style=Optimised  visibilities=8 + 1024 + 2^18 + 2^20  floatPrecision=float32_m23  warnSaturation=on  version=20211007  SampleTime=inf
  Convert : DSPBAPrim/Convert  primtype=convert  nInputs=1  nOutputs=1  omode=Specify via dialog  otype=ufix(1)  scale=0  rndmethod=Unbiased  factor=1  satmethod=None  shift_vec=[0 1 2 -1]  value=round([0:255]/17)  inPortNames=[' '; ' ';]  outPortNames=[' '; 'c']  dspbaimage=dspba_prim_wide.svg  text=fprintf('convert');  style=Optimised  visibilities=8+64+256+2^17  clipdetect=off  floatPrecision=float32_m23  advOptions=[]  version=20211007
  Finite State Machine : DSPBAUtilities/Finite State Machine  desc_file=fsm_control_falling_edge.fsm  latency=0  simulationMode=Bit And Cycle Accurate  finiteStateMachine=on
  GPIn : DSPBAPrim/GPIn  Commented=through  primtype=gpin  nInputs=evalAionMaskParam(gcb,'value',1)  nOutputs=evalAionMaskParam(gcb,'value',1)  omode=Inherit via internal rule  otype=sfix(16)  scale=2^-15  rndmethod=Unbiased  factor=1  satmethod=Symmetric  shift_vec=[0 1 2 -1]  value=1  inPortNames=[' ' ' ' ' ' ' ' ' ' ' ' ' ' ' ' ' ' ' ' ' ' ' ' ' ' ' ' ' ' ' ' ' ' ' ' ' ' ' ' ' ' ' ' ' ' ' ' ' ' ' ' ' ' ' ' ' ' ' ' ' ' ' ' ' ' ' ' ' ']'  outPortNames=[' ' ' ' ' ' ' ' ' ' ' ' ' ' ' ' ' ' ' ' ' ' ' ' ' ' ' ' ' ' ' ' ' ' ' ' ' ' ' ' ' ' ' ' ' ' ' ' ' ' ' ' ' ' ' ' ' ' ' ' ' ' ' ' ' ' ' ' ' ']'  dspbaimage=dspba_prim_channel_tall.svg  text=fprintf('GPIn%s', AdvDSPBInDisplay(latencyCorrection));  style=Optimised  visibilities=1024  latencyCorrection=0  scheduleOrigin=on  version=20211214
  GPOut : DSPBAPrim/GPOut  Commented=through  primtype=gpout  nInputs=evalAionMaskParam(gcb,'value',1)  nOutputs=evalAionMaskParam(gcb,'value',1)  omode=Inherit via internal rule  otype=sfix(16)  scale=2^-15  rndmethod=Unbiased  factor=1  satmethod=Symmetric  shift_vec=[0 1 2 -1]  value=1  inPortNames=[' ' ' ' ' ' ' ' ' ' ' ' ' ' ' ' ' ' ' ' ' ' ' ' ' ' ' ' ' ' ' ' ' ' ' ' ' ' ' ' ' ' ' ' ' ' ' ' ' ' ' ' ' ' ' ' ' ' ' ' ' ' ' ' ' ' ' ' ' ']'  outPortNames=[' ' ' ' ' ' ' ' ' ' ' ' ' ' ' ' ' ' ' ' ' ' ' ' ' ' ' ' ' ' ' ' ' ' ' ' ' ' ' ' ' ' ' ' ' ' ' ' ' ' ' ' ' ' ' ' ' ' ' ' ' ' ' ' ' ' ' ' ' ']'  dspbaimage=dspba_prim_channel_tall.svg  text=fprintf('GPOut%s', AdvDSPBOutDisplay(latency, latencyCorrection));  style=Optimised  visibilities=1024  latency=0  latencyCorrection=0  version=20211214
  SynthesisInfo : DSPBAPrim/SynthesisInfo  Commented=on  primtype=synthinfo  nInputs=0  nOutputs=0  omode=Inherit via internal rule  otype=sfix(16)  scale=2^-15  rndmethod=Truncate  factor=1  satmethod=Symmetric  shift_vec=[0 1 2 -1]  value=99  inPortNames=[' '; ' ';]  outPortNames=[' ']  dspbaimage=dspba_prim_ctrl.jpg  text=fprintf('Style=%s', style);  style=Scheduled  visibilities=2^17+2^18+2^19+2^20+2^21+2^22+2^23+2^24  constraintPair=GPIn to GPOut  constraintRelation==  constraintLimit=0  modelRefSign=+  modelRef=''  showSchedule=off  simulationMode=Use Global Value  resetMinimization=Conditional - On for ChannelIn/Out only  version=20220106
  falling_edge : Outport
  wires:
  GPIn/1 -> Convert/1
  Finite State Machine/1 -> GPOut/1
  Const/1 -> Finite State Machine/1
  GPOut/1 -> falling_edge/1
  in/1 -> GPIn/1
  Convert/1 -> Finite State Machine/2

== system lib_lowphy/iFFT_B2S ==
  data1 : Inport
  valid : Inport  Port=2
  channel1 : Inport  Port=3
  size1 : Inport  Port=4
  cplen1 : Inport  Port=5
  nsc1 : Inport  Port=6
  ifft_gain_re_l1 : Inport  Port=7
  ifft_gain_im_l1 : Inport  Port=8
  ifft_shift_l1 : Inport  Port=9
  ifft_mux_const_l1 : Inport  Port=10
  muxsel_l1 : Inport  Port=11
  DC_SC_EN : Inport  Port=12
  ripple_comp_en : Inport  Port=13
  rc_bw_sel : Inport  Port=14
  time_in : Inport  Port=15
  B2S : Subsystem
  IFFT : Subsystem
  To Workspace : ToWorkspace  Commented=on  VariableName=mod_vout  SaveFormat=Timeseries  SampleTime=-1
  To Workspace1 : ToWorkspace  Commented=on  VariableName=mod_cout  SaveFormat=Timeseries  SampleTime=-1
  To Workspace2 : ToWorkspace  Commented=on  VariableName=mod_dout  SaveFormat=Timeseries  SampleTime=-1
  vout1 : Outport
  cout1 : Outport  Port=2
  dout1 : Outport  Port=3
  td_ifft_out_d : Outport  Port=4
  td_ifft_out_ch : Outport  Port=5
  td_ifft_out_v : Outport  Port=6
  ifft_size_out : Outport  Port=7
  ifft_nprb_out : Outport  Port=8
  ifft_cp_out : Outport  Port=9
  fd_data_v : Outport  Port=10
  fd_data_c : Outport  Port=11
  fd_data_q : Outport  Port=12
  fd_time_out : Outport  Port=13
  wires:
  B2S/1(vout1) -> To Workspace/1, vout1/1
  cplen1/1 -> IFFT/5(cplen1)
  data1/1 -> IFFT/1(data1)
  valid/1 -> IFFT/2(valid1)
  ifft_gain_im_l1/1 -> IFFT/8(ifft_gain_im_l1)
  ifft_shift_l1/1 -> IFFT/9(ifft_shift_l1)
  DC_SC_EN/1 -> IFFT/12(DC_SC_EN)
  ifft_mux_const_l1/1 -> IFFT/10(ifft_mux_const_l1)
  size1/1 -> IFFT/4(size1)
  IFFT/3(dout1) -> B2S/3(q_in), td_ifft_out_d/1  "modified_fft_dout"
  channel1/1 -> IFFT/3(channel1)
  muxsel_l1/1 -> IFFT/11(muxsel_l1)
  nsc1/1 -> IFFT/6(nsc1)
  ifft_gain_re_l1/1 -> IFFT/7(ifft_gain_re_l1)
  IFFT/5(cpout1) -> B2S/5(cplen), ifft_cp_out/1
  IFFT/4(sizeout1) -> B2S/4(sizein), ifft_size_out/1
  B2S/3(dout1) -> To Workspace2/1, dout1/1
  IFFT/2(cout1) -> B2S/2(c_in), td_ifft_out_ch/1  "modified_fft_cout"
  IFFT/1(vout1) -> td_ifft_out_v/1, B2S/1(v_in)  "modified_fft_vout"
  B2S/2(cout1) -> To Workspace1/1, cout1/1
  IFFT/6(nprb) -> B2S/6(nprb), ifft_nprb_out/1
  ripple_comp_en/1 -> IFFT/13(ripple_comp_en)
  rc_bw_sel/1 -> IFFT/14(rc_bw_sel)
  IFFT/7(fd_data_v) -> fd_data_v/1
  IFFT/8(fd_data_c) -> fd_data_c/1
  IFFT/9(fd_data_q) -> fd_data_q/1
  IFFT/10(fd_time_out) -> fd_time_out/1
  time_in/1 -> IFFT/15(time_in)

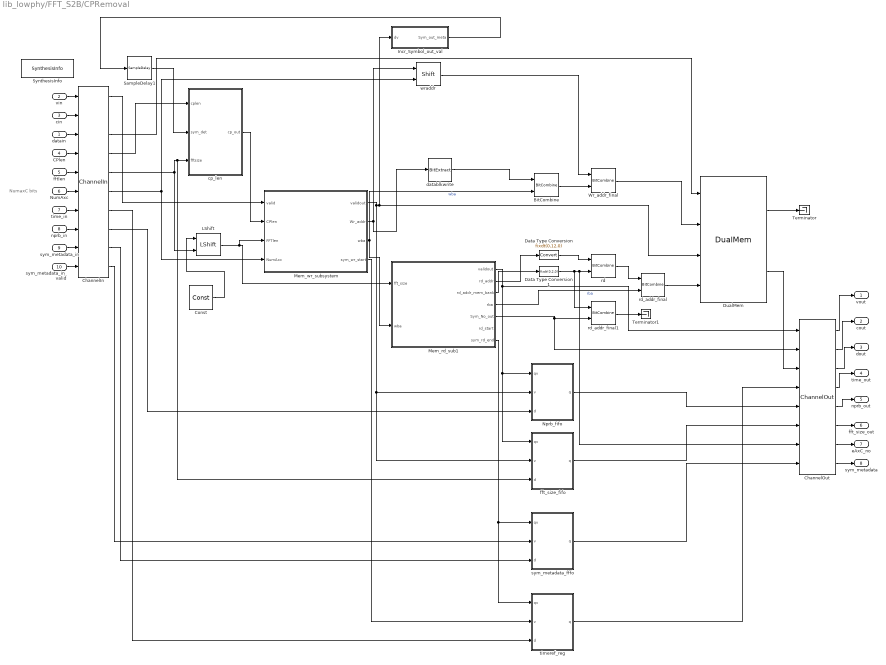
== system lib_lowphy/FFT_S2B/CPRemoval ==
  note: NumaxC bits
  datain : Inport
  vin : Inport  Port=2
  cin : Inport  Port=3
  CPlen : Inport  Port=4
  fftlen : Inport  Port=5
  NumAxc : Inport  Port=6
  time_in : Inport  Port=7
  nprb_in : Inport  Port=8
  sym_metadata_in : Inport  Port=9
  sym_metadata_in_valid : Inport  Port=10
  BitCombine : DSPBAPrim/BitCombine  primtype=bitcombine  nInputs=2  nOutputs=1  omode=Inherit via internal rule  otype=sfix(16)  scale=2^-15  rndmethod=Unbiased  factor=1  satmethod=Symmetric  shift_vec=[0 1 2 -1]  value=0  inPortNames=['l'; 'h';]  outPortNames=[' ']  dspbaimage=dspba_prim.svg  text=fprintf('[h,l]');  style=Optimised  visibilities=8+2  version=20211007
  ChannelIn : DSPBAPrim/ChannelIn  primtype=channelin  nInputs=dspba_internal_get_channel_ports(gcb)  nOutputs=dspba_internal_get_channel_ports(gcb)  omode=Inherit via internal rule  otype=sfix(16)  scale=2^-15  rndmethod=Unbiased  factor=1  satmethod=Symmetric  shift_vec=[0 1 2 -1]  value=8  inPortNames=['v'; 'c'; '0'; '1'; '2'; '3'; '4'; '5'; '6'; '7'; '8'; '9'; 'A'; 'B'; 'D'; 'E'; 'F'; 'G'; 'H'; 'I'; 'J'; 'K'; 'L'; 'M'; 'N'; 'O'; 'P'; 'Q'; 'R'; 'S'; 'T'; 'U'; 'W'; 'X'; 'Y'; 'Z']  outPortNames=['v'; 'c'; '0'; '1'; '2'; '3'; '4'; '5'; '6'; '7'; '8'; '9'; 'A'; 'B'; 'D'; 'E'; 'F'; 'G'; 'H'; 'I'; 'J'; 'K'; 'L'; 'M'; 'N'; 'O'; 'P'; 'Q'; 'R'; 'S'; 'T'; 'U'; 'W'; 'X'; 'Y'; 'Z']  dspbaimage=dspba_prim_channel_tall.svg  text=fprintf('In');  style=Optimised  dataSignals=8  foldingEnabled=off  channels=1  sampleRate=200  packetBeginPresent=off  packetBeginEnabled=off  visibilities=dspba_ChannelInVis(gcb)  latencyCorrection=0  scheduleOrigin=on  version=20211214
  ChannelOut : DSPBAPrim/ChannelOut  primtype=channelout  nInputs=dspba_internal_get_channel_ports(gcb)  nOutputs=dspba_internal_get_channel_ports(gcb)  omode=Inherit via internal rule  otype=sfix(16)  scale=2^-15  rndmethod=Unbiased  factor=1  satmethod=Symmetric  shift_vec=[0 1 2 -1]  value=6  inPortNames=['v'; 'c'; '0'; '1'; '2'; '3'; '4'; '5'; '6'; '7'; '8'; '9'; 'A'; 'B'; 'D'; 'E'; 'F'; 'G'; 'H'; 'I'; 'J'; 'K'; 'L'; 'M'; 'N'; 'O'; 'P'; 'Q'; 'R'; 'S'; 'T'; 'U'; 'W'; 'X'; 'Y'; 'Z']  outPortNames=['v'; 'c'; '0'; '1'; '2'; '3'; '4'; '5'; '6'; '7'; '8'; '9'; 'A'; 'B'; 'D'; 'E'; 'F'; 'G'; 'H'; 'I'; 'J'; 'K'; 'L'; 'M'; 'N'; 'O'; 'P'; 'Q'; 'R'; 'S'; 'T'; 'U'; 'W'; 'X'; 'Y'; 'Z']  dspbaimage=dspba_prim_channel_tall.svg  text=fprintf('Out%s', AdvDSPBChannelOutDisplay(latency));  style=Optimised  dataSignals=6  foldingEnabled=off  channels=1  sampleRate=200  packetBeginPresent=off  packetBeginEnabled=off  visibilities=dspba_ChannelOutVis(gcb)  latency=17  latencyCorrection=0  version=20211214
  Const : DSPBAPrim/Const  primtype=const  nInputs=0  nOutputs=1  omode=Specify via dialog  otype=fixdt(0,13,0)  scale=0  rndmethod=Unbiased  factor=1  satmethod=Symmetric  shift_vec=[0 1 2 -1]  value=1  inPortNames=['+'; '+';]  outPortNames=[' ']  dspbaimage=dspba_prim.svg  text=fprintf('%s', num2str(value));  style=Optimised  visibilities=8 + 1024  floatPrecision=float32_m23  warnSaturation=on  version=20211007  SampleTime=inf
  Data Type Conversion : DataTypeConversion  OutDataTypeStr=fixdt(0,12,0)  SaturateOnIntegerOverflow=off  RndMeth=Floor
  Data Type Conversion1 : DataTypeConversion  OutDataTypeStr=fixdt(0,2,0)  SaturateOnIntegerOverflow=off  RndMeth=Floor
  DualMem : DSPBAPrim/DualMem  primtype=dualmem  nInputs=4  nOutputs=2  omode=Inherit via internal rule  otype=sfix(16)  scale=2^-15  rndmethod=Unbiased  factor=1  satmethod=Symmetric  shift_vec=[0 1 2 -1]  value=[zeros(4096*4*2, 1)]  inPortNames=['d1'; 'a1'; 'w1'; 'd2'; 'a2'; 'w2']  outPortNames=['q1'; 'q2']  dspbaimage=dspba_prim_tall.svg  text=fprintf('dmem%s',AdvDSPBDMemDisplay(UseDontCare));  style=Optimised  visibilities=8 + 1024 + 2^17 + 2^18  UseDontCare=on  TwinWritePorts=off  init=on  ProvideReadAccess=off  version=20211007
  Incr_Symbol_out_val : Subsystem
  LShift : DSPBAPrim/LShift  primtype=lshift  nInputs=2  nOutputs=1  omode=Specify via dialog  otype=sfix(16)  scale=0  rndmethod=Unbiased  factor=1  satmethod=Symmetric  shift_vec=[0 1 2 -1]  value=0  inPortNames=['a'; 'b';]  outPortNames=[' ']  dspbaimage=dspba_prim.svg  text=fprintf('a << b');  style=Optimised  visibilities=8  version=20211007
  Mem_rd_sub1 : Subsystem
  Mem_wr_subsystem : Subsystem
  Nprb_fifo : Subsystem
  SampleDelay1 : DSPBAPrim/SampleDelay  primtype=sampdelay  nInputs=1  nOutputs=1  omode=Inherit via internal rule  otype=sfix(16)  scale=2^-15  rndmethod=Unbiased  factor=1  satmethod=Symmetric  shift_vec=[0 1 2 -1]  floatPrecision=float32_m23  value=4  inPortNames=[' '; ' ';]  outPortNames=[' ']  dspbaimage=dspba_prim.svg  text=dpoly(1, eye(1,value+1), 'z')  style=Optimised  visibilities=8 + 1024 + 2^17 + 2^18  flexible=off  slackgroup=0  augmented=3  version=20211007  advOptions=[]
  SynthesisInfo : DSPBAPrim/SynthesisInfo  primtype=synthinfo  nInputs=0  nOutputs=0  omode=Inherit via internal rule  otype=sfix(16)  scale=2^-15  rndmethod=Truncate  factor=1  satmethod=Symmetric  shift_vec=[0 1 2 -1]  value=99  inPortNames=[' '; ' ';]  outPortNames=[' ']  dspbaimage=dspba_prim_ctrl.jpg  text=fprintf('Style=%s', style);  style=Scheduled  visibilities=2^17+2^18+2^19+2^20+2^21+2^22+2^23+2^24  constraintPair=None  constraintRelation=>  constraintLimit=2  modelRefSign=+  modelRef=''  showSchedule=off  simulationMode=Use Global Value  resetMinimization=Conditional - On for ChannelIn/Out only  version=20220106
  Terminator : Terminator
  Terminator1 : Terminator
  Wr_addr_final : DSPBAPrim/BitCombine  primtype=bitcombine  nInputs=2  nOutputs=1  omode=Inherit via internal rule  otype=sfix(16)  scale=2^-15  rndmethod=Unbiased  factor=1  satmethod=Symmetric  shift_vec=[0 1 2 -1]  value=0  inPortNames=['l'; 'h';]  outPortNames=[' ']  dspbaimage=dspba_prim.svg  text=fprintf('[h,l]');  style=Optimised  visibilities=8+2  version=20211007
  cp_len : Subsystem
  datablkwrite : DSPBAPrim/BitExtract  primtype=bitextract  nInputs=1  nOutputs=1  omode=Specify via dialog  otype=fixdt(0,2,0)  scale=1  rndmethod=Unbiased  factor=1  satmethod=Symmetric  shift_vec=[0 1 2 -1]  value=0  inPortNames=[' '; ' ';]  outPortNames=[' ']  dspbaimage=dspba_prim.svg  text=fprintf('..%d', value);  style=Optimised  visibilities=8+1024  version=20211007
  fft_size_fifo : Subsystem
  rd : DSPBAPrim/BitCombine  primtype=bitcombine  nInputs=2  nOutputs=1  omode=Inherit via internal rule  otype=sfix(16)  scale=2^-15  rndmethod=Unbiased  factor=1  satmethod=Symmetric  shift_vec=[0 1 2 -1]  value=0  inPortNames=['l'; 'h';]  outPortNames=[' ']  dspbaimage=dspba_prim.svg  text=fprintf('[h,l]');  style=Optimised  visibilities=8+2  version=20211007
  rd_addr_final : DSPBAPrim/BitCombine  primtype=bitcombine  nInputs=2  nOutputs=1  omode=Inherit via internal rule  otype=sfix(16)  scale=2^-15  rndmethod=Unbiased  factor=1  satmethod=Symmetric  shift_vec=[0 1 2 -1]  value=0  inPortNames=['l'; 'h';]  outPortNames=[' ']  dspbaimage=dspba_prim.svg  text=fprintf('[h,l]');  style=Optimised  visibilities=8+2  version=20211007
  rd_addr_final1 : DSPBAPrim/BitCombine  primtype=bitcombine  nInputs=2  nOutputs=1  omode=Inherit via internal rule  otype=sfix(16)  scale=2^-15  rndmethod=Unbiased  factor=1  satmethod=Symmetric  shift_vec=[0 1 2 -1]  value=0  inPortNames=['l'; 'h';]  outPortNames=[' ']  dspbaimage=dspba_prim.svg  text=fprintf('[h,l]');  style=Optimised  visibilities=8+2  version=20211007
  sym_metadata_fffo : Subsystem
  timeref_reg : Subsystem
  wraddr : DSPBAPrim/Shift  primtype=shift  nInputs=2  nOutputs=1  omode=Specify via dialog  otype=fixdt(0,12,0)  scale=0  rndmethod=Unbiased  factor=1  satmethod=Symmetric  shift_vec=[0 1 2 -1]  value=0  inPortNames=['a'; 'b';]  outPortNames=[' ']  dspbaimage=dspba_prim.svg  text=fprintf('a >> b');  style=Optimised  visibilities=8  version=20211007
  "vout " : Outport
  cout : Outport  Port=2
  dout : Outport  Port=3
  time_out : Outport  Port=4
  nprb_out : Outport  Port=5
  fft_size_out : Outport  Port=6
  eAxC_no : Outport  Port=7
  sym_metadata : Outport  Port=8
  wires:
  Mem_rd_sub1/1(validout) -> Nprb_fifo/1(qv), fft_size_fifo/1(qv), ChannelOut/1
  ChannelIn/6 -> wraddr/2, Mem_wr_subsystem/4(NumAxc)
  ChannelIn/5 -> fft_size_fifo/3(d), cp_len/3(fftsize), LShift/2
  Data Type Conversion1/1 -> rd_addr_final1/1, ChannelOut/7, rd/2
  vin/1 -> ChannelIn/1
  ChannelOut/3 -> dout/1
  ChannelIn/1 -> Mem_wr_subsystem/1(valid)
  BitCombine/1 -> Wr_addr_final/2
  Mem_wr_subsystem/3(wba) -> Mem_rd_sub1/2(wba), BitCombine/2  "wba"
  wraddr/1 -> Wr_addr_final/1
  Mem_rd_sub1/4(rba) -> rd_addr_final/2  "rba"
  rd_addr_final/1 -> DualMem/4
  LShift/1 -> Mem_wr_subsystem/3(FFTlen), Mem_rd_sub1/1(fft_size)
  Mem_rd_sub1/5(Sym_No_out) -> ChannelOut/2, rd_addr_final1/2
  DualMem/2 -> ChannelOut/3
  ChannelIn/3 -> DualMem/1
  SampleDelay1/1 -> cp_len/2(sym_det)
  Nprb_fifo/1(q) -> ChannelOut/5
  Mem_wr_subsystem/2(Wr_addr) -> datablkwrite/1, wraddr/1
  ChannelIn/4 -> cp_len/1(cplen)
  datain/1 -> ChannelIn/3
  ChannelOut/5 -> nprb_out/1
  ChannelOut/4 -> time_out/1
  cp_len/1(cp_out) -> Mem_wr_subsystem/2(CPlen)
  Incr_Symbol_out_val/1(Sym_out_meta) -> SampleDelay1/1
  rd_addr_final1/1 -> Terminator1/1
  ChannelIn/8 -> Nprb_fifo/3(d)
  ChannelOut/1 -> "vout "/1
  ChannelOut/2 -> cout/1
  nprb_in/1 -> ChannelIn/8
  ChannelOut/6 -> fft_size_out/1
  fft_size_fifo/1(q) -> ChannelOut/6
  time_in/1 -> ChannelIn/7
  cin/1 -> ChannelIn/2
  Data Type Conversion/1 -> rd/1
  Wr_addr_final/1 -> DualMem/2
  Const/1 -> LShift/1
  Mem_wr_subsystem/1(validout) -> Nprb_fifo/2(v), fft_size_fifo/2(v), DualMem/3, Incr_Symbol_out_val/1(dv)
  rd/1 -> rd_addr_final/1
  NumAxc/1 -> ChannelIn/6
  DualMem/1 -> Terminator/1
  datablkwrite/1 -> BitCombine/1
  Mem_rd_sub1/2(rd_addr) -> Data Type Conversion/1
  CPlen/1 -> ChannelIn/4
  Mem_rd_sub1/3(rd_addr_mem_bank) -> Data Type Conversion1/1
  fftlen/1 -> ChannelIn/5
  sym_metadata_in/1 -> ChannelIn/9
  sym_metadata_in_valid/1 -> ChannelIn/10
  ChannelOut/7 -> eAxC_no/1
  ChannelOut/8 -> sym_metadata/1
  sym_metadata_fffo/1(q) -> ChannelOut/8
  timeref_reg/1(q) -> ChannelOut/4
  Mem_rd_sub1/7(sym_rd_end) -> timeref_reg/1(qv), sym_metadata_fffo/1(qv)
  ChannelIn/7 -> timeref_reg/3(d)
  ChannelIn/9 -> sym_metadata_fffo/3(d)
  ChannelIn/10 -> sym_metadata_fffo/2(v)
  Mem_wr_subsystem/4(sym_wr_start) -> timeref_reg/2(v)
